simulink model "Lextue18_BodyModel"  (R2017b)
settings: Solver=VariableStepAuto  StartTime=0.0  StopTime=10.0  RelTol=1e-3
undefined symbols (not defined in the file): g, m1
settings Model: Creator=jtb32  LastModifiedBy=jtb32

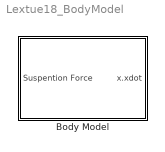
== system Lextue18_BodyModel ==
  Body Model : Subsystem

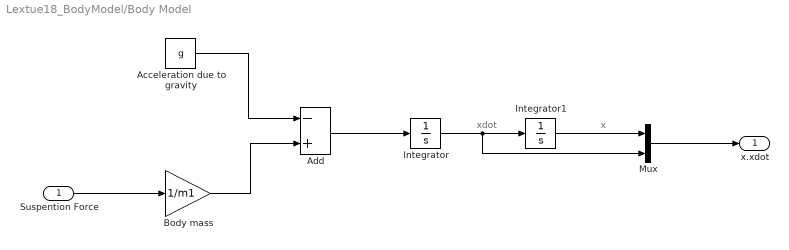
== system Lextue18_BodyModel/Body Model ==
  note: xdot
  note: x
  "Suspention Force " : Inport
  Acceleration due to gravity : Constant  Value=g
  Add : Sum  Inputs=-+
  Body mass : Gain  Gain=1/m1
  Integrator : Integrator
  Integrator1 : Integrator
  Mux : Mux  Inputs=2
  x.xdot : Outport
  wires:
  Body mass/1 -> Add/2
  Integrator/1 -> Mux/2, Integrator1/1
  Add/1 -> Integrator/1
  Acceleration due to gravity/1 -> Add/1
  Integrator1/1 -> Mux/1
  "Suspention Force "/1 -> Body mass/1
  Mux/1 -> x.xdot/1
